simulink model "ConveyorSpeedControlSystem"  (R2025b)
settings: Solver=FixedStepAuto  StartTime=0.0  StopTime=30  FixedStep=0.01  RelTol=1e-3
libraries: slpidlib x1, simulink x1
settings Model: Creator=anpan  LastModifiedBy=anpan

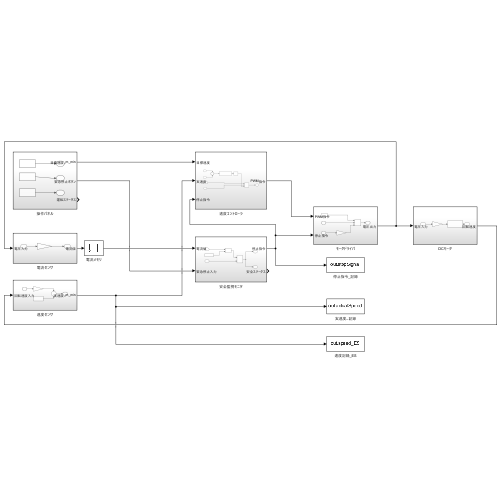
[thumbnail: Simulink's stored preview of the top-level diagram]
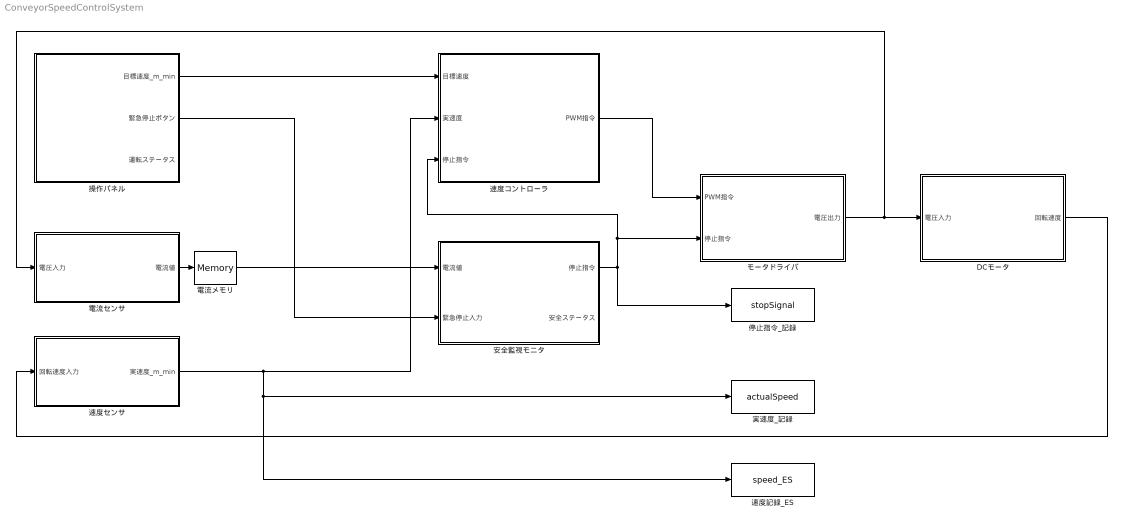
== system ConveyorSpeedControlSystem ==
  DCモータ : Subsystem
  モータドライバ : Subsystem
  停止指令_記録 : ToWorkspace  VariableName=stopSignal  SaveFormat=Timeseries  SampleTime=0.01
  安全監視モニタ : Subsystem
  実速度_記録 : ToWorkspace  VariableName=actualSpeed  SaveFormat=Timeseries  SampleTime=0.01
  操作パネル : Subsystem
  速度コントローラ : Subsystem
  速度センサ : Subsystem
  速度記録_ES : ToWorkspace  VariableName=speed_ES  SaveFormat=Timeseries  SampleTime=0.01
  電流センサ : Subsystem
  電流メモリ : Memory
  wires:
  操作パネル/1(目標速度_m_min) -> 速度コントローラ/1(目標速度)
  操作パネル/2(緊急停止ボタン) -> 安全監視モニタ/2(緊急停止入力)
  安全監視モニタ/1(停止指令) -> 速度コントローラ/3(停止指令), モータドライバ/2(停止指令), 停止指令_記録/1
  速度コントローラ/1(PWM指令) -> モータドライバ/1(PWM指令)
  モータドライバ/1(電圧出力) -> 電流センサ/1(電圧入力), DCモータ/1(電圧入力)
  DCモータ/1(回転速度) -> 速度センサ/1(回転速度入力)
  速度センサ/1(実速度_m_min) -> 実速度_記録/1, 速度記録_ES/1, 速度コントローラ/2(実速度)
  電流センサ/1(電流値) -> 電流メモリ/1
  電流メモリ/1 -> 安全監視モニタ/1(電流値)

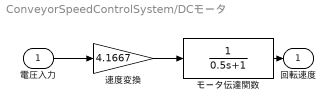
== system ConveyorSpeedControlSystem/DCモータ ==
  電圧入力 : Inport
  モータ伝達関数 : TransferFcn  Denominator=[0.5 1]
  速度変換 : Gain  Gain=4.1667
  回転速度 : Outport
  wires:
  電圧入力/1 -> 速度変換/1
  速度変換/1 -> モータ伝達関数/1
  モータ伝達関数/1 -> 回転速度/1

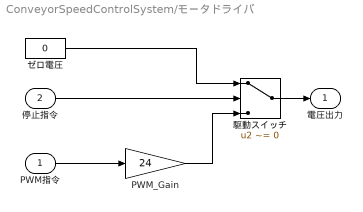
== system ConveyorSpeedControlSystem/モータドライバ ==
  PWM指令 : Inport
  停止指令 : Inport  Port=2
  PWM_Gain : Gain  Gain=24
  ゼロ電圧 : Constant  Value=0
  駆動スイッチ : Switch  Criteria=u2 ~= 0
  電圧出力 : Outport
  wires:
  PWM指令/1 -> PWM_Gain/1
  停止指令/1 -> 駆動スイッチ/2
  駆動スイッチ/1 -> 電圧出力/1
  ゼロ電圧/1 -> 駆動スイッチ/1
  PWM_Gain/1 -> 駆動スイッチ/3

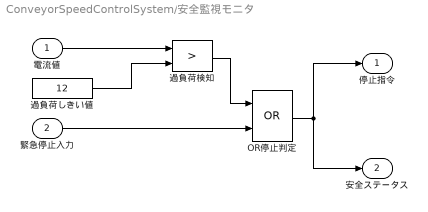
== system ConveyorSpeedControlSystem/安全監視モニタ ==
  電流値 : Inport
  緊急停止入力 : Inport  Port=2
  OR停止判定 : Logic  Operator=OR  AllPortsSameDT=off  OutDataTypeStr=boolean
  過負荷しきい値 : Constant  Value=12
  過負荷検知 : RelationalOperator  Operator=>  OutDataTypeStr=boolean  RndMeth=Simplest  InputSameDT=off
  停止指令 : Outport
  安全ステータス : Outport  Port=2
  wires:
  電流値/1 -> 過負荷検知/1
  過負荷しきい値/1 -> 過負荷検知/2
  過負荷検知/1 -> OR停止判定/1
  緊急停止入力/1 -> OR停止判定/2
  OR停止判定/1 -> 停止指令/1, 安全ステータス/1

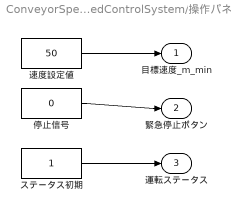
== system ConveyorSpeedControlSystem/操作パネル ==
  ステータス初期 : Constant
  停止信号 : Constant  Value=0
  速度設定値 : Constant  Value=50
  目標速度_m_min : Outport
  緊急停止ボタン : Outport  Port=2
  運転ステータス : Outport  Port=3
  wires:
  速度設定値/1 -> 目標速度_m_min/1
  ステータス初期/1 -> 運転ステータス/1
  停止信号/1 -> 緊急停止ボタン/1

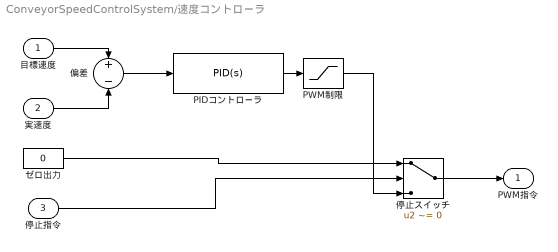
== system ConveyorSpeedControlSystem/速度コントローラ ==
  目標速度 : Inport
  実速度 : Inport  Port=2
  停止指令 : Inport  Port=3
  PIDコントローラ : slpidlib/PID Controller  Controller=PID  Form=Parallel  TimeDomain=Continuous-time  UseExternalTs=off  SampleTime=-1  IntegratorMethod=Forward Euler  FilterMethod=Forward Euler  ControllerParametersSource=internal  P=0.10  I=0.040  UseKiTs=off  D=0.005  UseExternalDerivativeSource=off  N=100  UseFilter=on  TunerSelectOption=Transfer Function Based (PID Tuner App)  InitialConditionSource=internal  InitialConditionForIntegrator=0  InitialConditionForFilter=0  DifferentiatorICPrevScaledInput=0  ExternalReset=none  TrackingMode=off  Kt=1  LimitOutput=off  SatLimitsSource=internal  UpperSaturationLimit=inf  LowerSaturationLimit=-inf  LinearizeAsGain=on  AntiWindupMode=none  Kb=1  LimitIntegrator=off  UpperIntegratorSaturationLimit=inf  LowerIntegratorSaturationLimit=-inf  POutMin=[]  POutMax=[]  IOutMin=[]  IOutMax=[]  DOutMin=[]  DOutMax=[]  NOutMin=[]  NOutMax=[]  SumOutMin=[]  SumOutMax=[]  SaturationOutMin=[]  SaturationOutMax=[]  PParamMin=[]  PParamMax=[]  IParamMin=[]  IParamMax=[]  DParamMin=[]  DParamMax=[]  NParamMin=[]  NParamMax=[]  KbParamMin=[]  KbParamMax=[]  KtParamMin=[]  KtParamMax=[]  KbOutMin=[]  KbOutMax=[]  KtOutMin=[]  KtOutMax=[]  IntegratorOutMin=[]  IntegratorOutMax=[]  FilterOutMin=[]  FilterOutMax=[]  SumI1OutMin=[]  SumI1OutMax=[]  SumI2OutMin=[]  SumI2OutMax=[]  SumI3OutMin=[]  SumI3OutMax=[]  SumI4OutMin=[]  SumI4OutMax=[]  SumDOutMin=[]  SumDOutMax=[]  DifferentiatorOutMin=[]  DifferentiatorOutMax=[]  FilterDiffOutCoefMin=[]  FilterDiffOutCoefMax=[]  ReciprocalOutMin=[]  ReciprocalOutMax=[]  SumDenOutMin=[]  SumDenOutMax=[]  SumNumOutMin=[]  SumNumOutMax=[]  DivideOutMin=[]  DivideOutMax=[]  UdiffTsProdOutMin=[]  UdiffTsProdOutMax=[]  NTsProdOutMin=[]  NTsProdOutMax=[]  UintegralTsProdOutMin=[]  UintegralTsProdOutMax=[]  UngainTsProdOutMin=[]  UngainTsProdOutMax=[]  ClampingZeroOutDataTypeStr=Inherit: Inherit via back propagation  ClampingZeroOutMin=[]  ClampingZeroOutMax=[]  FilterDenConstantOutDataTypeStr=Inherit: Inherit via back propagation  FilterDenConstantOutMin=[]  FilterDenConstantOutMax=[]  PCopyOutDataTypeStr=Inherit: Inherit via back propagation  PCopyOutMin=[]  PCopyOutMax=[]  NCopyOutDataTypeStr=Inherit: Inherit via back propagation  NCopyOutMin=[]  NCopyOutMax=[]  IntegratorContinuousStateAttributes=''  IntegratorStateMustResolveToSignalObject=off  IntegratorRTWStateStorageClass=Auto  FilterContinuousStateAttributes=''  FilterStateMustResolveToSignalObject=off  FilterRTWStateStorageClass=Auto  ParallelPVariant=InternalParameters  IdealPVariant=Disabled  IVariant=InternalParameters  DVariant=InternalParameters  IntegratorVariant=Continuous  SatVariant=Disabled  AWVariant=Passthrough  PCopyVariant=Disabled  TRVariant=Disabled  FdbkBlocksVariant=Forward  IdealPFdbkVariant=Disabled  SatFdbkVariant=Disabled  DerivativeFilterVariant=ContFilter  NVariant=InternalParameters  NCopyVariant=Disabled  FilterICVariant=InternalICsFilter  IntegratorICVariant=InternalICs  ExternalResetVariant=Disabled  TRSumVariant=Passthrough  SumFdbkVariant=Disabled  SumVariant=Sum_PID  TsampFilterVariant=InternalTs  TsampNgainVariant=Passthrough  TsampIntegralVariant=Disabled_SignalSpec  ExternalSaturationOutDataTypeStr=Inherit: Same as second input  DerivativeSourceVariant=ErrorSignal  PreIntVariant=InternalPreInt
  PWM制限 : Saturate  UpperLimit=1  LowerLimit=0
  ゼロ出力 : Constant  Value=0
  偏差 : Sum  Inputs=+-
  停止スイッチ : Switch  Criteria=u2 ~= 0
  PWM指令 : Outport
  wires:
  目標速度/1 -> 偏差/1
  実速度/1 -> 偏差/2
  偏差/1 -> PIDコントローラ/1
  停止指令/1 -> 停止スイッチ/2
  停止スイッチ/1 -> PWM指令/1
  ゼロ出力/1 -> 停止スイッチ/1
  PIDコントローラ/1 -> PWM制限/1
  PWM制限/1 -> 停止スイッチ/3

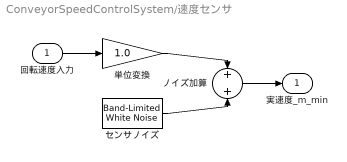
== system ConveyorSpeedControlSystem/速度センサ ==
  回転速度入力 : Inport
  センサノイズ : simulink/Sources/Band-Limited White Noise  Cov=0.01  Ts=0.1  seed=[23341]
  ノイズ加算 : Sum
  単位変換 : Gain  Gain=1.0
  実速度_m_min : Outport
  wires:
  回転速度入力/1 -> 単位変換/1
  単位変換/1 -> ノイズ加算/1
  センサノイズ/1 -> ノイズ加算/2
  ノイズ加算/1 -> 実速度_m_min/1

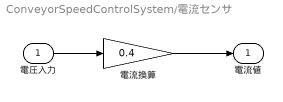
== system ConveyorSpeedControlSystem/電流センサ ==
  電圧入力 : Inport
  電流換算 : Gain  Gain=0.4
  電流値 : Outport
  wires:
  電圧入力/1 -> 電流換算/1
  電流換算/1 -> 電流値/1
